simulink model "Control_no_duty"  (R2021a)
settings: Solver=VariableStepAuto  StartTime=0.0  StopTime=10  RelTol=1e-3
values from neighbouring files (symbols this model uses):
  Calc_delay = 20e-6    (= 2e-05)    [Control.m]
  J = 0.00052*1000    (= 0.52)    [Control.m]
  Kf = 0.1*10    (= 1)    [Control.m]
  Ki = double(vpasolve(num(3)==Ki/Lq,Ki))    [Control.m]
  Kp = double(vpasolve(num(2)==Rq/Lq+Kp/Lq,Kp))    [Control.m]
  lambda = 0.032    [Control.m]
  Ld = Lq    (= 5.25e-05)    [Control.m]
  Lq = 0.0525*10^-3    (= 5.25e-05)    [Control.m]
  Rd = 0.013/2    (= 0.0065)    [Control.m]
  Rq = Rd    (= 0.0065)    [Control.m]
  Ts = 1/Fsw    (= 9.3808630394e-05)    [Control.m]
  Vbat = 14.4*4    (= 57.6)    [Control.m]
libraries: mcbcontrolslib x8
settings Model: Creator=jacob  LastModifiedBy=jacob

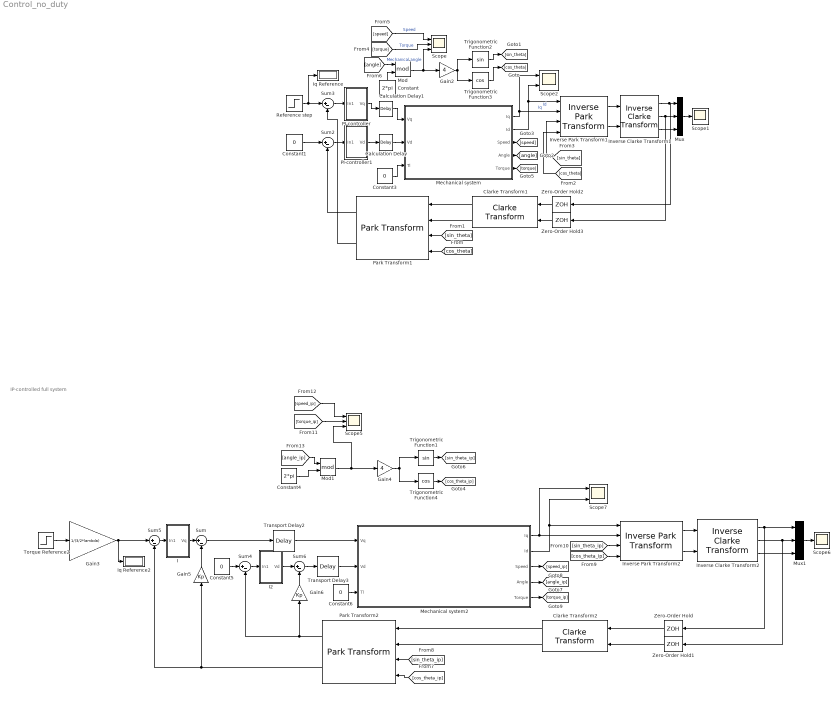
== system Control_no_duty ==
  note: IP-controlled full system
  Calculation Delay : TransportDelay  DelayTime=Calc_delay
  Calculation Delay1 : TransportDelay  DelayTime=Calc_delay
  Clarke Transform1 : mcbcontrolslib/Clarke Transform  VariantControl=Variant2
  Clarke Transform2 : mcbcontrolslib/Clarke Transform  VariantControl=Variant2
  Constant : Constant  Value=2*pi
  Constant{1,3,5..6} (4 alike) : Constant  Value=0
  Constant4 : Constant  Value=2*pi
  Gain2 : Gain  Gain=4
  Gain3 : Gain  Gain=1/(3/2*lambda)
  Gain4 : Gain  Gain=4
  Gain5 : Gain  Gain=Kp
  Gain6 : Gain  Gain=Kp
  I : Subsystem
  I2 : Subsystem
  Inverse Clarke Transform1 : mcbcontrolslib/Inverse Clarke Transform
      settings: SourceProductBaseCode=MT
  Inverse Clarke Transform2 : mcbcontrolslib/Inverse Clarke Transform
      settings: SourceProductBaseCode=MT
  Inverse Park Transform1 : mcbcontrolslib/Inverse Park Transform  AxisAlignment=D-axis
  Inverse Park Transform2 : mcbcontrolslib/Inverse Park Transform  AxisAlignment=D-axis
  Iq Reference : Display
      settings: Decimation=3
  Iq Reference2 : Display
      settings: Decimation=3
  Mechanical system : Subsystem
  Mechanical system2 : Subsystem
  Mod : Math  Operator=mod  SaturateOnIntegerOverflow=on
  Mod1 : Math  Operator=mod  SaturateOnIntegerOverflow=on
  Mux : Mux  Inputs=3
  Mux1 : Mux  Inputs=3
  PI-controller : Subsystem
  PI-controller1 : Subsystem
  Park Transform1 : mcbcontrolslib/Park Transform  AxisAlignment=D-axis
      settings: SourceProductBaseCode=MT
  Park Transform2 : mcbcontrolslib/Park Transform  AxisAlignment=D-axis
      settings: SourceProductBaseCode=MT
  Reference step : Step  Time=0.1  After=311  SampleTime=0
  Scope : Scope  NumInputPorts=3
  Scope1 : Scope
  Scope2 : Scope  NumInputPorts=2
  Scope5 : Scope  NumInputPorts=3
  Scope6 : Scope
  Scope7 : Scope  NumInputPorts=2
  Sum{,2..6} (6 alike) : Sum  Inputs=|+-
  Torque Reference2 : Step  Time=0.1  After=15  SampleTime=0
  Transport Delay2 : TransportDelay  DelayTime=Calc_delay
  Transport Delay3 : TransportDelay  DelayTime=Calc_delay
  Trigonometric Function1 : Trigonometry
  Trigonometric Function2 : Trigonometry
  Trigonometric Function3 : Trigonometry  Operator=cos
  Trigonometric Function4 : Trigonometry  Operator=cos
  Zero-Order Hold{,1..3} (4 alike) : ZeroOrderHold  SampleTime=Ts
  wires:
  Mechanical system/1(Iq) -> Inverse Park Transform1/2, Scope2/1  "Iq"
  Mechanical system/2(Id) -> Inverse Park Transform1/1, Scope2/2  "Id"
  Trigonometric Function3/1 -> [cos_theta]
  Trigonometric Function2/1 -> [sin_theta]
  Inverse Park Transform1/1 -> Inverse Clarke Transform1/1
  Inverse Park Transform1/2 -> Inverse Clarke Transform1/2
  Inverse Clarke Transform1/1 -> Zero-Order Hold2/1, Mux/1
  Inverse Clarke Transform1/2 -> Mux/2, Zero-Order Hold3/1
  Clarke Transform1/1 -> Park Transform1/1
  Clarke Transform1/2 -> Park Transform1/2
  Sum3/1 -> PI-controller/1(In1)
  Park Transform1/2 -> Sum3/2
  Sum2/1 -> PI-controller1/1(In1)
  Park Transform1/1 -> Sum2/2
  Gain2/1 -> Trigonometric Function3/1, Trigonometric Function2/1
  Mux/1 -> Scope1/1
  Inverse Clarke Transform1/3 -> Mux/3
  Constant1/1 -> Sum2/1
  Reference step/1 -> Iq Reference/1, Sum3/1
  Constant3/1 -> Mechanical system/3(Tl)
  [sin_theta] -> Inverse Park Transform1/3
  [cos_theta] -> Inverse Park Transform1/4
  [sin_theta] -> Park Transform1/3
  [cos_theta] -> Park Transform1/4
  Mechanical system/5(Torque) -> [torque]
  Mechanical system/4(Angle) -> [angle]
  Mechanical system/3(Speed) -> [speed]
  [torque] -> Scope/2  "Torque"
  [speed] -> Scope/1  "Speed"
  [angle] -> Mod/1
  Mod/1 -> Scope/3, Gain2/1  "Mechanical angle"
  Constant/1 -> Mod/2
  Constant6/1 -> Mechanical system2/3(Tl)
  Park Transform2/2 -> Gain5/1, Sum5/2
  Mechanical system2/3(Speed) -> [speed_ip]
  Mod1/1 -> Scope5/3, Gain4/1
  [cos_theta_ip] -> Park Transform2/4
  Inverse Park Transform2/1 -> Inverse Clarke Transform2/1
  Sum5/1 -> I/1(In1)
  Mechanical system2/5(Torque) -> [torque_ip]
  Inverse Clarke Transform2/2 -> Zero-Order Hold1/1, Mux1/2
  Constant4/1 -> Mod1/2
  Gain4/1 -> Trigonometric Function4/1, Trigonometric Function1/1
  Constant5/1 -> Sum4/1
  Mux1/1 -> Scope6/1
  [cos_theta_ip] -> Inverse Park Transform2/4
  [torque_ip] -> Scope5/2
  Inverse Clarke Transform2/3 -> Mux1/3
  Torque Reference2/1 -> Gain3/1
  [sin_theta_ip] -> Inverse Park Transform2/3
  Mechanical system2/4(Angle) -> [angle_ip]
  [sin_theta_ip] -> Park Transform2/3
  [speed_ip] -> Scope5/1
  Clarke Transform2/1 -> Park Transform2/1
  Trigonometric Function1/1 -> [sin_theta_ip]
  Inverse Park Transform2/2 -> Inverse Clarke Transform2/2
  Mechanical system2/1(Iq) -> Inverse Park Transform2/2, Scope7/1
  Sum4/1 -> I2/1(In1)
  [angle_ip] -> Mod1/1
  Clarke Transform2/2 -> Park Transform2/2
  Trigonometric Function4/1 -> [cos_theta_ip]
  Inverse Clarke Transform2/1 -> Zero-Order Hold/1, Mux1/1
  Park Transform2/1 -> Gain6/1, Sum4/2
  Gain3/1 -> Sum5/1, Iq Reference2/1
  Mechanical system2/2(Id) -> Inverse Park Transform2/1, Scope7/2
  I/1(Vq) -> Sum/1
  Gain5/1 -> Sum/2
  I2/1(Vd) -> Sum6/1
  Gain6/1 -> Sum6/2
  PI-controller/1(Vq) -> Calculation Delay1/1
  Calculation Delay1/1 -> Mechanical system/1(Vq)
  PI-controller1/1(Vd) -> Calculation Delay/1
  Calculation Delay/1 -> Mechanical system/2(Vd)
  Transport Delay2/1 -> Mechanical system2/1(Vq)
  Sum/1 -> Transport Delay2/1
  Sum6/1 -> Transport Delay3/1
  Zero-Order Hold1/1 -> Clarke Transform2/2
  Zero-Order Hold/1 -> Clarke Transform2/1
  Zero-Order Hold3/1 -> Clarke Transform1/2
  Zero-Order Hold2/1 -> Clarke Transform1/1
  Transport Delay3/1 -> Mechanical system2/2(Vd)

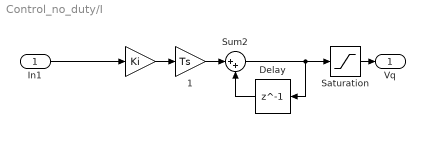
== system Control_no_duty/I ==
  In1 : Inport
  " " : Gain  Gain=Ki
  " 1" : Gain  Gain=Ts
  Delay : Delay  DelayLength=1  SampleTime=Ts
  Saturation : Saturate  UpperLimit=Vbat  LowerLimit=-Vbat
  Sum2 : Sum  Inputs=|++
  Vq : Outport
  wires:
  " 1"/1 -> Sum2/1
  Delay/1 -> Sum2/2
  " "/1 -> " 1"/1
  In1/1 -> " "/1
  Sum2/1 -> Delay/1, Saturation/1
  Saturation/1 -> Vq/1

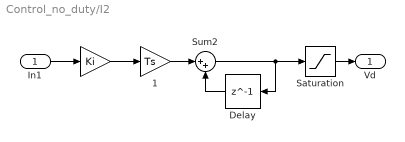
== system Control_no_duty/I2 ==
  In1 : Inport
  " " : Gain  Gain=Ki
  " 1" : Gain  Gain=Ts
  Delay : Delay  DelayLength=1  SampleTime=Ts
  Saturation : Saturate  UpperLimit=Vbat  LowerLimit=-Vbat
  Sum2 : Sum  Inputs=|++
  Vd : Outport
  wires:
  " 1"/1 -> Sum2/1
  Delay/1 -> Sum2/2
  " "/1 -> " 1"/1
  In1/1 -> " "/1
  Saturation/1 -> Vd/1
  Sum2/1 -> Delay/1, Saturation/1

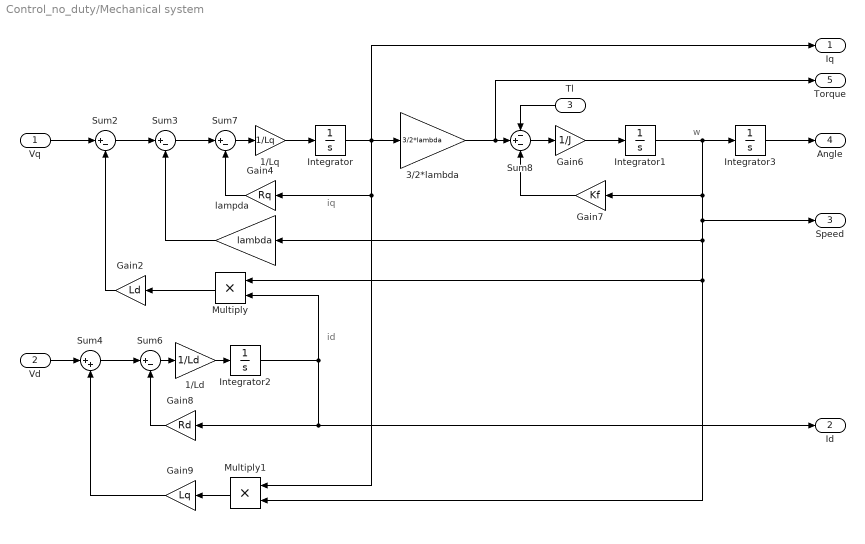
== system Control_no_duty/Mechanical system ==
  note: iq
  note: w
  note: id
  Vq : Inport
  Vd : Inport  Port=2
  Tl : Inport  Port=3
  1/Ld : Gain  Gain=1/Ld
  1/Lq : Gain  Gain=1/Lq
  3/2*lambda : Gain  Gain=3/2*lambda
  Gain2 : Gain  Gain=Ld
  Gain4 : Gain  Gain=Rq
  Gain6 : Gain  Gain=1/J
  Gain7 : Gain  Gain=Kf
  Gain8 : Gain  Gain=Rd
  Gain9 : Gain  Gain=Lq
  Integrator{,1..3} (4 alike) : Integrator
  Multiply : Product
  Multiply1 : Product
  Sum{2..3,6..7} (4 alike) : Sum  Inputs=|+-
  Sum4 : Sum  Inputs=|++
  Sum8 : Sum  Inputs=-+-
  lampda : Gain  Gain=lambda
  Iq : Outport
  Id : Outport  Port=2
  Speed : Outport  Port=3
  Angle : Outport  Port=4
  Torque : Outport  Port=5
  wires:
  Gain4/1 -> Sum7/2
  Sum2/1 -> Sum3/1
  Gain6/1 -> Integrator1/1
  Sum7/1 -> 1/Lq/1
  Vd/1 -> Sum4/1
  Sum6/1 -> 1/Ld/1
  Sum4/1 -> Sum6/1
  lampda/1 -> Sum3/2
  1/Lq/1 -> Integrator/1
  Gain2/1 -> Sum2/2
  Integrator2/1 -> Id/1, Gain8/1, Multiply/2
  Integrator1/1 -> Integrator3/1, Speed/1, Multiply1/2, Multiply/1, lampda/1, Gain7/1
  Sum8/1 -> Gain6/1
  Integrator/1 -> 3/2*lambda/1, Gain4/1, Multiply1/1, Iq/1
  Integrator3/1 -> Angle/1
  Multiply1/1 -> Gain9/1
  Gain9/1 -> Sum4/2
  Gain8/1 -> Sum6/2
  1/Ld/1 -> Integrator2/1
  Sum3/1 -> Sum7/1
  Multiply/1 -> Gain2/1
  Vq/1 -> Sum2/1
  3/2*lambda/1 -> Sum8/2, Torque/1
  Gain7/1 -> Sum8/3
  Tl/1 -> Sum8/1

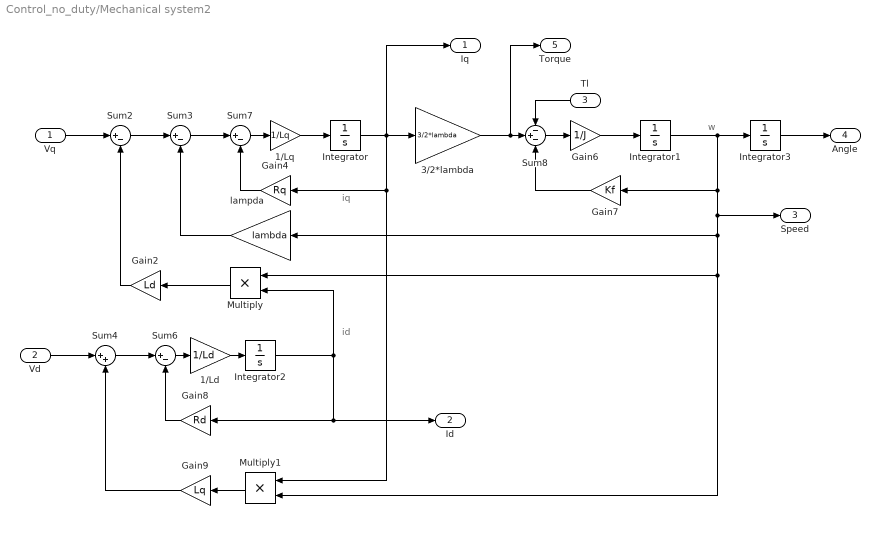
== system Control_no_duty/Mechanical system2 ==
  note: iq
  note: w
  note: id
  Vq : Inport
  Vd : Inport  Port=2
  Tl : Inport  Port=3
  1/Ld : Gain  Gain=1/Ld
  1/Lq : Gain  Gain=1/Lq
  3/2*lambda : Gain  Gain=3/2*lambda
  Gain2 : Gain  Gain=Ld
  Gain4 : Gain  Gain=Rq
  Gain6 : Gain  Gain=1/J
  Gain7 : Gain  Gain=Kf
  Gain8 : Gain  Gain=Rd
  Gain9 : Gain  Gain=Lq
  Integrator{,1..3} (4 alike) : Integrator
  Multiply : Product
  Multiply1 : Product
  Sum{2..3,6..7} (4 alike) : Sum  Inputs=|+-
  Sum4 : Sum  Inputs=|++
  Sum8 : Sum  Inputs=-+-
  lampda : Gain  Gain=lambda
  Iq : Outport
  Id : Outport  Port=2
  Speed : Outport  Port=3
  Angle : Outport  Port=4
  Torque : Outport  Port=5
  wires:
  Gain4/1 -> Sum7/2
  Sum2/1 -> Sum3/1
  Gain6/1 -> Integrator1/1
  Sum7/1 -> 1/Lq/1
  Vd/1 -> Sum4/1
  Sum6/1 -> 1/Ld/1
  Sum4/1 -> Sum6/1
  lampda/1 -> Sum3/2
  1/Lq/1 -> Integrator/1
  Gain2/1 -> Sum2/2
  Integrator2/1 -> Id/1, Gain8/1, Multiply/2
  Integrator1/1 -> Integrator3/1, Speed/1, Multiply1/2, Multiply/1, lampda/1, Gain7/1
  Sum8/1 -> Gain6/1
  Integrator/1 -> 3/2*lambda/1, Gain4/1, Multiply1/1, Iq/1
  Integrator3/1 -> Angle/1
  Multiply1/1 -> Gain9/1
  Gain9/1 -> Sum4/2
  Gain8/1 -> Sum6/2
  1/Ld/1 -> Integrator2/1
  Sum3/1 -> Sum7/1
  Multiply/1 -> Gain2/1
  Vq/1 -> Sum2/1
  3/2*lambda/1 -> Sum8/2, Torque/1
  Gain7/1 -> Sum8/3
  Tl/1 -> Sum8/1

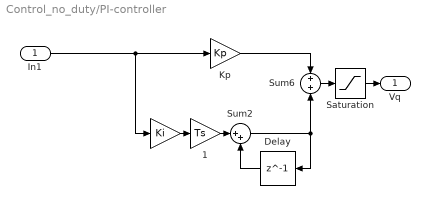
== system Control_no_duty/PI-controller ==
  In1 : Inport
  " " : Gain  Gain=Ki
  " 1" : Gain  Gain=Ts
  Delay : Delay  DelayLength=1  SampleTime=Ts
  Kp : Gain  Gain=Kp
  Saturation : Saturate  UpperLimit=Vbat  LowerLimit=-Vbat
  Sum2 : Sum  Inputs=|++
  Sum6 : Sum  Inputs=+|+
  Vq : Outport
  wires:
  " 1"/1 -> Sum2/1
  Delay/1 -> Sum2/2
  Kp/1 -> Sum6/1
  " "/1 -> " 1"/1
  Sum2/1 -> Delay/1, Sum6/2
  In1/1 -> " "/1, Kp/1
  Sum6/1 -> Saturation/1
  Saturation/1 -> Vq/1

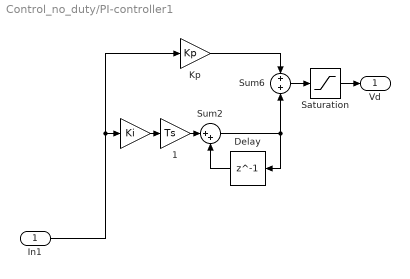
== system Control_no_duty/PI-controller1 ==
  In1 : Inport
  " " : Gain  Gain=Ki
  " 1" : Gain  Gain=Ts
  Delay : Delay  DelayLength=1  SampleTime=Ts
  Kp : Gain  Gain=Kp
  Saturation : Saturate  UpperLimit=Vbat  LowerLimit=-Vbat
  Sum2 : Sum  Inputs=|++
  Sum6 : Sum  Inputs=+|+
  Vd : Outport
  wires:
  " 1"/1 -> Sum2/1
  Delay/1 -> Sum2/2
  Kp/1 -> Sum6/1
  " "/1 -> " 1"/1
  Sum2/1 -> Delay/1, Sum6/2
  In1/1 -> Kp/1, " "/1
  Saturation/1 -> Vd/1
  Sum6/1 -> Saturation/1
